simulink model "single_panel_mppt_lookup_sim"  (R2021b)
settings: Solver=ode23tb  StartTime=0.0  StopTime=sim_time  FixedStep=5e-5  MaxStep=max_time_step  RelTol=1e-3
values from neighbouring files (symbols this model uses):
  actions = (-1:1) * duty_step    [single_panel_mppt_lookup.m]
  alpha = 0.1    [single_panel_mppt_lookup.m]
  deg_threshold = deg2rad(5)    [single_panel_mppt_lookup.m]
  exploration_factor_init = 0.9999    [single_panel_mppt_lookup.m]
  gamma = 0.9    [single_panel_mppt_lookup.m]
  Irradiance = 1000    [single_panel_mppt_lookup.m]
  Isc = 5.17    [single_panel_mppt_lookup.m]
  n_I = 100    [single_panel_mppt_lookup.m]
  n_V = 100    [single_panel_mppt_lookup.m]
  Ts = 1e-3    (= 0.001)    [single_panel_mppt_lookup.m]
  Voc = 43.99    [single_panel_mppt_lookup.m]
  wn = 4    [single_panel_mppt_lookup.m]
  wp = 1    [single_panel_mppt_lookup.m]
undefined symbols (not defined in the file or in its folder): current, irr_data, mpp_data, voltage
libraries: simulink x2, spspowerguiLib x1
settings Model: Creator=HP  LastModifiedBy=HP

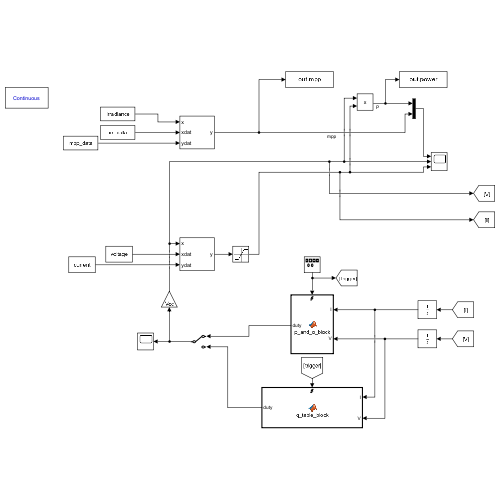
[thumbnail: Simulink's stored preview of the top-level diagram]
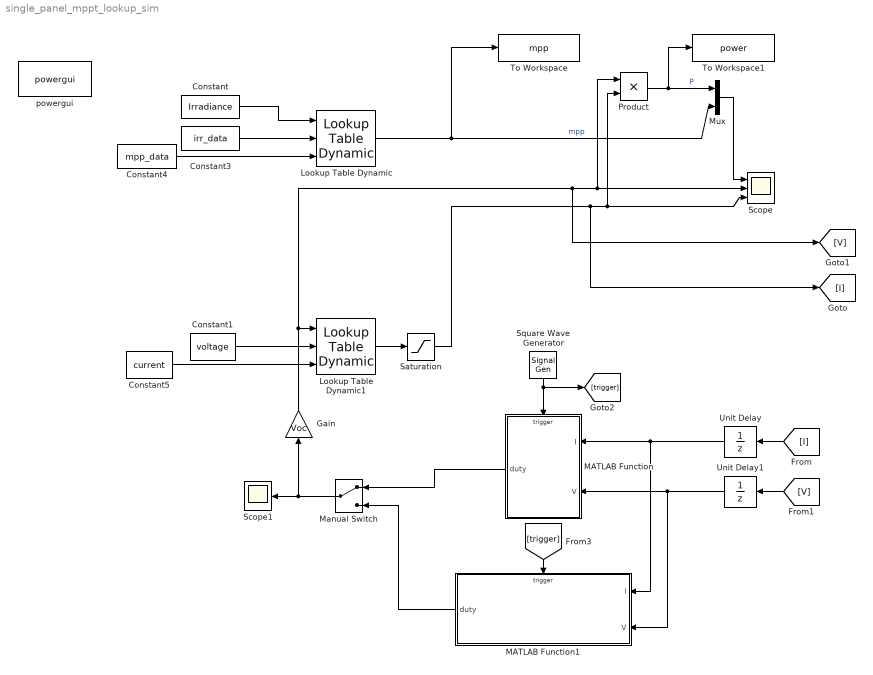
== system single_panel_mppt_lookup_sim ==
  Constant : Constant  Value=Irradiance
  Constant1 : Constant  Value=voltage
  Constant3 : Constant  Value=irr_data
  Constant4 : Constant  Value=mpp_data
  Constant5 : Constant  Value=current
  Gain : Gain  Gain=Voc
  Lookup Table Dynamic : simulink/Lookup Tables/Lookup Table Dynamic  LookUpMeth=Interpolation-Use End Values  OutDataType=fixdt('double')  OutScaling=[]  OutputDataTypeScalingMode=Specify via dialog  OutDataTypeStr=double  DoSatur=off
  Lookup Table Dynamic1 : simulink/Lookup Tables/Lookup Table Dynamic  LookUpMeth=Interpolation-Use End Values  OutDataType=fixdt('double')  OutScaling=[]  OutputDataTypeScalingMode=Specify via dialog  OutDataTypeStr=double  DoSatur=off
  MATLAB Function : MATLAB Function  TreatAsAtomicUnit=on
  MATLAB Function1 : MATLAB Function  TreatAsAtomicUnit=on
  Manual Switch : ManualSwitch
  Mux : Mux  Inputs=2
  Product : Product
  Saturation : Saturate  UpperLimit=Isc  LowerLimit=0
  Scope : Scope  NumInputPorts=3
  Scope1 : Scope
  Square Wave Generator : SignalGenerator  WaveForm=square  Frequency=1/Ts
  To Workspace : ToWorkspace  VariableName=mpp  SaveFormat=Timeseries  SampleTime=-1
  To Workspace1 : ToWorkspace  VariableName=power  SaveFormat=Timeseries  SampleTime=-1
  Unit Delay : UnitDelay  SampleTime=-1  HasFrameUpgradeWarning=on
  Unit Delay1 : UnitDelay  SampleTime=-1  HasFrameUpgradeWarning=on
  powergui : spspowerguiLib/powergui  Priority=1  SimulationMode=Continuous  SampleTime=50e-6  frequency=60  Iterations=50  frequencyindice=0  Pbase=100e6  ErrMax=1e-4  UnitsV=kV  UnitsW=MW  buscounter=0  FunctionMessages=off  echomessages=off  EnableUseOfTLC=off  CurrentSourceSwitches=off  DisableSnubberDevices=off  DisableRonSwitches=off  DisableVfSwitches=off  DisplayEquations=off  AutomaticDiscreteSolvers=off  SolverType=Tustin/Backward Euler (TBE)  Interpol=off  ExternalGateDelay=off  methode=off  Ts=100  x0status=blocks  SPID=on  SwTol=0  HookPort=off  NonlinearTolerance=1e-4  nMaxIteration=100  ContinueOnMaxIteration=off  RestoreLinks=warning  ResistiveCurrentMeasurement=off  Frange=[0:2:500]  Ylog=off  Xlog=on  ShowGrid=off  save=off  variable=ZData  structure=0  ZoomFFT=off  StartTime=0.0  cycles=1  DisplayStyle=1  fundamental=60  FreqAxis=off  MaxFrequency=1000  frequencyindicesteady=1  RmsSteady=1  display=off
  wires:
  Gain/1 -> [V], Product/1, Scope/2, Lookup Table Dynamic1/1
  Lookup Table Dynamic1/1 -> Saturation/1
  [I] -> Unit Delay/1
  [V] -> Unit Delay1/1
  Product/1 -> To Workspace1/1, Mux/1  "P"
  Mux/1 -> Scope/1
  Lookup Table Dynamic/1 -> To Workspace/1, Mux/2  "mpp"
  Constant3/1 -> Lookup Table Dynamic/2
  Constant4/1 -> Lookup Table Dynamic/3
  Square Wave Generator/1 -> MATLAB Function/Trigger, [trigger]
  [trigger] -> MATLAB Function1/Trigger
  Unit Delay1/1 -> MATLAB Function1/2(V), MATLAB Function/2(V)
  Unit Delay/1 -> MATLAB Function1/1(I), MATLAB Function/1(I)
  MATLAB Function/1(duty) -> Manual Switch/1
  MATLAB Function1/1(duty) -> Manual Switch/2
  Manual Switch/1 -> Scope1/1, Gain/1
  Constant5/1 -> Lookup Table Dynamic1/3
  Constant1/1 -> Lookup Table Dynamic1/2
  Constant/1 -> Lookup Table Dynamic/1
  Saturation/1 -> [I], Scope/3, Product/2

== matlab function single_panel_mppt_lookup_sim/MATLAB Function ==
  data: I input; duty output; V input; duty_step parameter
  events: trigger input RISING_EDGE_EVENT
% @p_and_o - a function implementing the Perturb and Observe MPPT algorithm
function duty = p_and_o_block(I, V, duty_step)

    % make sure that function is included in the project path
    duty = 0; % a requried init so that the program knows the size of the var
    duty = p_and_o(I, V, duty_step);    
end

== matlab function single_panel_mppt_lookup_sim/MATLAB Function1 ==
  data: I input; duty output; V input; Voc parameter; Isc parameter; deg_threshold parameter; wp parameter; wn parameter; n_V parameter; n_I parameter; actions parameter; alpha parameter; gamma parameter; exploration_factor_init parameter
  events: trigger input RISING_EDGE_EVENT
function duty = q_table_block(I, V, Voc, Isc, deg_threshold, wp, wn, n_V, n_I, actions, alpha, gamma, exploration_factor_init)
    
    % make sure that function is included in the project path
    
    duty = 0; % a requried init so that the program knows the size of the var
    duty = q_table(I, V, Voc, Isc, deg_threshold, wp, wn, n_V, n_I, actions, alpha, gamma, exploration_factor_init);
end
